simulink model "Sistema"  (R2023a)
settings: Solver=ode15s  StartTime=0.0  StopTime=10.0  MaxStep=1E-3  RelTol=1e-3
libraries: fl_lib x12, nesl_utility x6, ee_lib x2, slpidlib x1
settings Model: LastModifiedBy=osiri
settings DataIOCC: SaveFormat=Array  ReturnWorkspaceOutputs=off  TimeSaveName=t
settings DebuggingCC: AlgebraicLoopMsg=none  ArtificialAlgebraicLoopMsg=none  MaxConsecutiveZCsMsg=none  ModelReferenceExtraNoncontSigs=none  OperatingPointInterfaceChecksumMismatchMsg=none
settings RTWCC: GPUComputeCapability=5.0

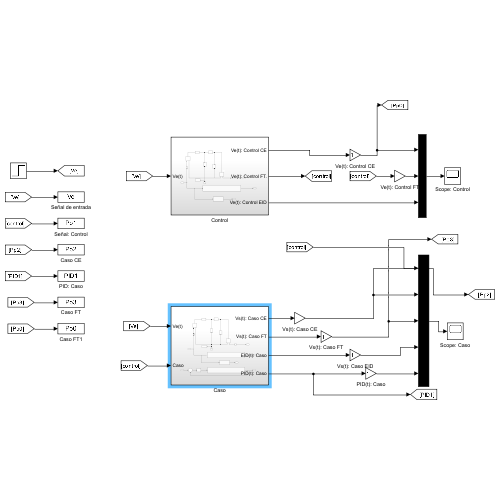
[thumbnail: Simulink's stored preview of the top-level diagram]
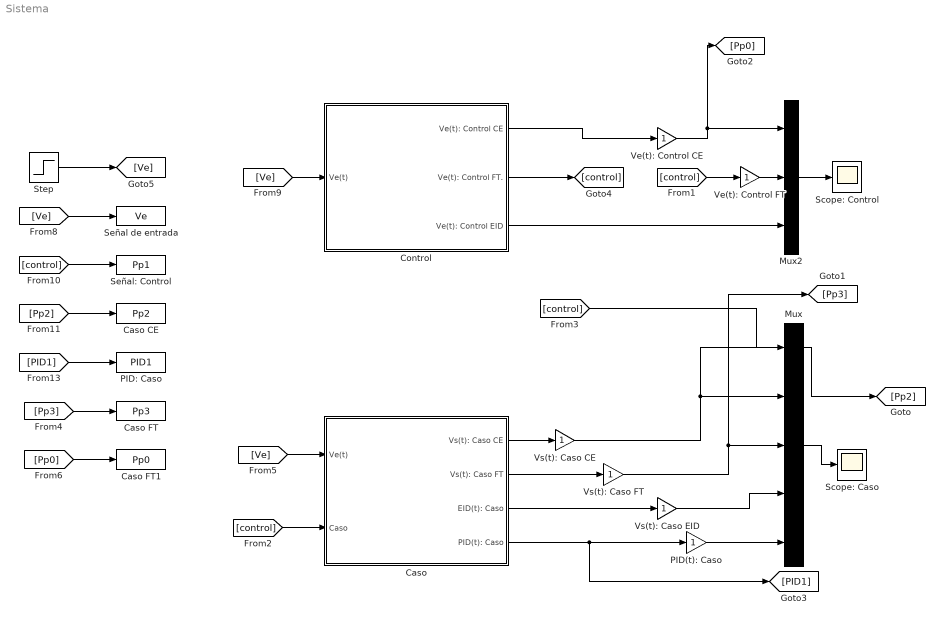
== system Sistema ==
  Caso : Subsystem
  Caso CE : ToWorkspace  VariableName=Pp2  SampleTime=-1
  Caso FT : ToWorkspace  VariableName=Pp3  SampleTime=-1
  Caso FT1 : ToWorkspace  VariableName=Pp0  SampleTime=-1
  Control : Subsystem
  Mux : Mux  Inputs=5
  Mux2 : Mux  Inputs=3
  PID(t): Caso : Gain
  PID: Caso : ToWorkspace  VariableName=PID1  SampleTime=-1
  Scope: Caso : Scope
  Scope: Control : Scope
  Señal de entrada : ToWorkspace  VariableName=Ve  SampleTime=-1
  Señal: Control : ToWorkspace  VariableName=Pp1  SampleTime=-1
  Step : Step  SampleTime=0
  Ve(t): Control CE : Gain
  Ve(t): Control FT : Gain
  Vs(t): Caso CE : Gain
  Vs(t): Caso EID : Gain
  Vs(t): Caso FT : Gain
  wires:
  Mux/1 -> Scope: Caso/1
  [control] -> Caso/2(Caso)
  [control] -> Mux/1
  Control/2(Ve(t): Control FT.) -> [control]
  Control/1(Ve(t): Control CE) -> Ve(t): Control CE/1
  Mux2/1 -> Scope: Control/1
  [Ve] -> Control/1(Ve(t))
  [control] -> Ve(t): Control FT/1
  [Ve] -> Señal de entrada/1
  [control] -> Señal: Control/1
  [Pp2] -> Caso CE/1
  [PID1] -> PID: Caso/1
  Step/1 -> [Ve]
  Ve(t): Control FT/1 -> Mux2/2
  Ve(t): Control CE/1 -> [Pp0], Mux2/1
  Vs(t): Caso CE/1 -> [Pp2], Mux/2
  Caso/1(Vs(t): Caso CE) -> Vs(t): Caso CE/1
  Vs(t): Caso FT/1 -> Mux/3, [Pp3]
  Caso/2(Vs(t): Caso FT) -> Vs(t): Caso FT/1
  Caso/4(PID(t): Caso) -> PID(t): Caso/1, [PID1]
  [Pp3] -> Caso FT/1
  [Pp0] -> Caso FT1/1
  Control/3(Ve(t): Control EID) -> Mux2/3
  PID(t): Caso/1 -> Mux/5
  Vs(t): Caso EID/1 -> Mux/4
  Caso/3(EID(t): Caso) -> Vs(t): Caso EID/1
  [Ve] -> Caso/1(Ve(t))

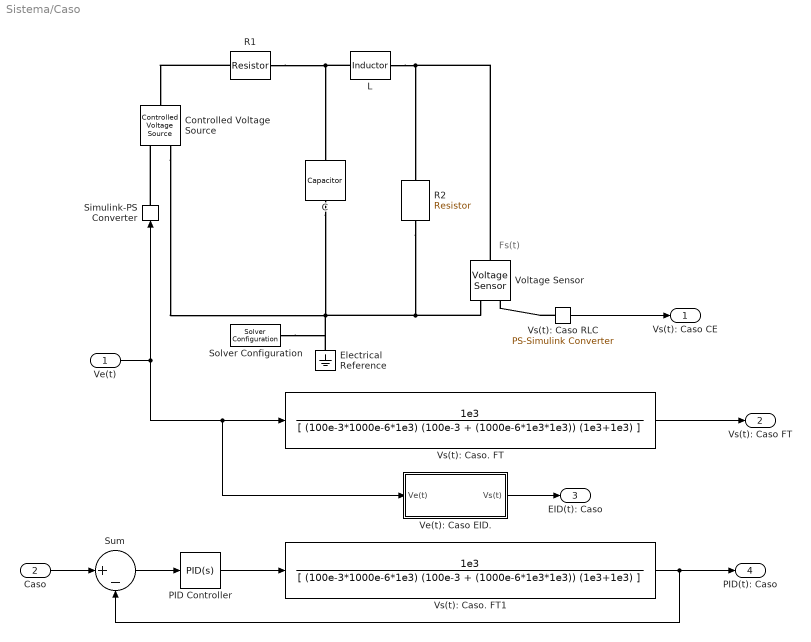
== system Sistema/Caso ==
  note: Fs(t)
  Ve(t) : Inport
  Caso : Inport  Port=2
  C : fl_lib/Electrical/Electrical Elements/Capacitor  c=1000e-6 F  r=1e-6 Ohm  g=0 1/Ohm  i_specify=off  i_priority=None  i=0 A  i_nominal_specify=off  i_nominal_unit=A  i_nominal_value=1  v_specify=off  v_priority=None  v=0 V  v_nominal_specify=off  v_nominal_unit=V  v_nominal_value=1  vc_specify=off  vc_priority=High  vc=0 V  vc_nominal_specify=off  vc_nominal_unit=V  vc_nominal_value=1
  Controlled Voltage Source : fl_lib/Electrical/Electrical Sources/Controlled Voltage Source
  Electrical Reference : fl_lib/Electrical/Electrical Elements/Electrical Reference
  L : ee_lib/Passive/Inductor  l=100e-3 H  enable_L_tol=ee.enum.toleranceApplication.none  L_tol=20  tol_distribution=ee.enum.toleranceDistribution.uniform  nSigma=4  r=0 Ohm  g=1e-9 1/Ohm  enable_operating_limits=ee.enum.enable.no  operating_limit_action=ee.enum.passive.reportOpLim.warn  max_working_current=1 A  power_rating=1 W  enable_faults=ee.enum.enable.no  fault_action=simscape.enum.assert.action.none  lambdaPercent=50  k_faulted=0.9999  turnsShort=ee.enum.passive.inductor.turnsShortOption.no  openCct=ee.enum.enable.no  groundShort=ee.enum.passive.inductor.groundShortOption.no  groundShortG=0 1/Ohm  tau_fault=1e-3 s  fault_trigger=ee.enum.faults.faultTrigger.temporal  t_fault=1 s  max_permissible_voltage=100 V  n_fail_on_voltage=1  max_permissible_current=1 A  t_fail_on_current=1 s  i_L_specify=off  i_L_priority=High  i_L=0 A  i_L_nominal_specify=off  i_L_nominal_unit=A  i_L_nominal_value=1
  PID Controller : slpidlib/PID Controller  Controller=PID  Form=Parallel  TimeDomain=Continuous-time  UseExternalTs=off  SampleTime=-1  IntegratorMethod=Forward Euler  FilterMethod=Forward Euler  ControllerParametersSource=internal  P=132.81296326735  I=3266.13831963624  UseKiTs=off  D=0.180716891182534  N=507.693883251119  UseFilter=on  TunerSelectOption=Transfer Function Based (PID Tuner App)  InitialConditionSource=internal  InitialConditionForIntegrator=0  InitialConditionForFilter=0  DifferentiatorICPrevScaledInput=0  ExternalReset=none  TrackingMode=off  Kt=1  LimitOutput=off  SatLimitsSource=internal  UpperSaturationLimit=inf  LowerSaturationLimit=-inf  LinearizeAsGain=on  AntiWindupMode=none  Kb=1  LimitIntegrator=off  UpperIntegratorSaturationLimit=inf  LowerIntegratorSaturationLimit=-inf  POutMin=[]  POutMax=[]  IOutMin=[]  IOutMax=[]  DOutMin=[]  DOutMax=[]  NOutMin=[]  NOutMax=[]  SumOutMin=[]  SumOutMax=[]  SaturationOutMin=[]  SaturationOutMax=[]  PParamMin=[]  PParamMax=[]  IParamMin=[]  IParamMax=[]  DParamMin=[]  DParamMax=[]  NParamMin=[]  NParamMax=[]  KbParamMin=[]  KbParamMax=[]  KtParamMin=[]  KtParamMax=[]  KbOutMin=[]  KbOutMax=[]  KtOutMin=[]  KtOutMax=[]  IntegratorOutMin=[]  IntegratorOutMax=[]  FilterOutMin=[]  FilterOutMax=[]  SumI1OutMin=[]  SumI1OutMax=[]  SumI2OutMin=[]  SumI2OutMax=[]  SumI3OutMin=[]  SumI3OutMax=[]  SumI4OutMin=[]  SumI4OutMax=[]  SumDOutMin=[]  SumDOutMax=[]  DifferentiatorOutMin=[]  DifferentiatorOutMax=[]  FilterDiffOutCoefMin=[]  FilterDiffOutCoefMax=[]  ReciprocalOutMin=[]  ReciprocalOutMax=[]  SumDenOutMin=[]  SumDenOutMax=[]  SumNumOutMin=[]  SumNumOutMax=[]  DivideOutMin=[]  DivideOutMax=[]  UdiffTsProdOutMin=[]  UdiffTsProdOutMax=[]  NTsProdOutMin=[]  NTsProdOutMax=[]  UintegralTsProdOutMin=[]  UintegralTsProdOutMax=[]  UngainTsProdOutMin=[]  UngainTsProdOutMax=[]  ClampingZeroOutDataTypeStr=Inherit: Inherit via back propagation  ClampingZeroOutMin=[]  ClampingZeroOutMax=[]  FilterDenConstantOutDataTypeStr=Inherit: Inherit via back propagation  FilterDenConstantOutMin=[]  FilterDenConstantOutMax=[]  PCopyOutDataTypeStr=Inherit: Inherit via back propagation  PCopyOutMin=[]  PCopyOutMax=[]  NCopyOutDataTypeStr=Inherit: Inherit via back propagation  NCopyOutMin=[]  NCopyOutMax=[]  IntegratorContinuousStateAttributes=''  IntegratorStateMustResolveToSignalObject=off  IntegratorRTWStateStorageClass=Auto  FilterContinuousStateAttributes=''  FilterStateMustResolveToSignalObject=off  FilterRTWStateStorageClass=Auto  ParallelPVariant=InternalParameters  IdealPVariant=Disabled  IVariant=InternalParameters  DVariant=InternalParameters  IntegratorVariant=Continuous  SatVariant=Disabled  AWVariant=Passthrough  PCopyVariant=Disabled  TRVariant=Disabled  FdbkBlocksVariant=Forward  IdealPFdbkVariant=Disabled  SatFdbkVariant=Disabled  DerivativeFilterVariant=ContFilter  NVariant=InternalParameters  NCopyVariant=Disabled  FilterICVariant=InternalICsFilter  IntegratorICVariant=InternalICs  ExternalResetVariant=Disabled  TRSumVariant=Passthrough  SumFdbkVariant=Disabled  SumVariant=Sum_PID  TsampFilterVariant=InternalTs  TsampNgainVariant=Passthrough  TsampIntegralVariant=Disabled_SignalSpec  ExternalSaturationOutDataTypeStr=Inherit: Same as second input
  R1 : fl_lib/Electrical/Electrical Elements/Resistor  R=1e3 Ohm  i_specify=off  i_priority=None  i=0 A  i_nominal_specify=off  i_nominal_unit=A  i_nominal_value=1  v_specify=off  v_priority=None  v=0 V  v_nominal_specify=off  v_nominal_unit=V  v_nominal_value=1
  R2 : fl_lib/Electrical/Electrical Elements/Resistor  R=1e3 Ohm  i_specify=off  i_priority=None  i=0 A  i_nominal_specify=off  i_nominal_unit=A  i_nominal_value=1  v_specify=off  v_priority=None  v=0 V  v_nominal_specify=off  v_nominal_unit=V  v_nominal_value=1
  Simulink-PS Converter : nesl_utility/Simulink-PS Converter  PhysicalDomain=network_engine_domain  SubClassName=ps_input  LeftPortType=input  RightPortType=output  PseudoPeriodic=off  Frequencies=[]  NoiseDistribution=none  NoiseParameters=[]  Unit=1  AffineConversion=off  FilteringAndDerivatives=provide  SimscapeFilterOrder=1  InputFilterTimeConstant=0.001  UdotUserProvided=0
  Solver Configuration : nesl_utility/Solver Configuration  PhysicalDomain=network_engine_domain  SubClassName=solver  LeftPortType=input  RightPortType=generic  Tones=[]  Harmonics=[]  SimulateNoise=off  Profile=off  UseLocalSampling=off  EnableSwitchedLinearOptims=on  FrequencyDomain=off  UseCCode=off  RelTol=0.001  AbsTol=0.001  MinStep=1e-09  ToWorkspace=off  RevertToSquareIcSolve=off  NumHomotopyIterations=100  PhasorMode=off  PhasorModeNumHarmonics=1  ConsistencySolver=NEWTON_XTOL_AFTER_FTOL  IndexReductionMethod=DerivativeReplacement  DoDC=off  ResidualTolerance=1e-09  ConsistencyTolSource=GLOBAL  ConsistencyAbsTol=0.001  ConsistencyRelTol=0.001  ConsistencyTolFactor=0.001  UseLocalSolver=off  LocalSolverChoice=NE_BACKWARD_EULER_ADVANCER  ResolveIndetEquations=on  FunctionEvalNumThread=1  LocalSolverSampleTime=0.001  DoFixedCost=off  MaxNonlinIter=3  MaxModeIter=2  ComputeImpulses=off  ImpulseIterations=2  LinearAlgebra=auto  LinearAlgebraNumThread=0  EquationFormulation=NE_TIME_EF  DelaysMemoryBudget=1024  AutomaticFiltering=on  FilteringTimeConstant=0.001  PartitionStorageMethod=AS_NEEDED  PartitionMemoryBudget=1024  PartitionMethod=ROBUST
  Sum : Sum  Inputs=|+-
  Ve(t): Caso EID. : Subsystem
  Voltage Sensor : fl_lib/Electrical/Electrical Sensors/Voltage Sensor
  Vs(t): Caso RLC : nesl_utility/PS-Simulink Converter  PhysicalDomain=network_engine_domain  SubClassName=ps_output  LeftPortType=input  RightPortType=output  PseudoPeriodic=off  Frequencies=[]  VectorFormat=1-D array  Unit=inherit  AffineConversion=off
  Vs(t): Caso. FT : TransferFcn  Numerator=[1e3]  Denominator=[ (100e-3*1000e-6*1e3) (100e-3 + (1000e-6*1e3*1e3)) (1e3+1e3) ]
  Vs(t): Caso. FT1 : TransferFcn  Numerator=[1e3]  Denominator=[ (100e-3*1000e-6*1e3) (100e-3 + (1000e-6*1e3*1e3)) (1e3+1e3) ]
  Vs(t): Caso CE : Outport
  Vs(t): Caso FT : Outport  Port=2
  EID(t): Caso : Outport  Port=3
  PID(t): Caso : Outport  Port=4
  wires:
  Sum/1 -> PID Controller/1
  Vs(t): Caso. FT1/1 -> PID(t): Caso/1, Sum/2
  PID Controller/1 -> Vs(t): Caso. FT1/1
  Caso/1 -> Sum/1
  Vs(t): Caso RLC/1 -> Vs(t): Caso CE/1
  Ve(t)/1 -> Ve(t): Caso EID./1(Ve(t)), Vs(t): Caso. FT/1, Simulink-PS Converter/1
  Vs(t): Caso. FT/1 -> Vs(t): Caso FT/1
  Ve(t): Caso EID./1(Vs(t)) -> EID(t): Caso/1
  connections:
  R1/LConn1 -- C/LConn1 -- L/LConn1
  Voltage Sensor/RConn2 -- Solver Configuration/RConn1 -- Electrical Reference/LConn1 -- C/RConn1 -- Controlled Voltage Source/RConn2 -- R2/LConn1
  Simulink-PS Converter/RConn1 -- Controlled Voltage Source/RConn1
  R1/RConn1 -- Controlled Voltage Source/LConn1
  Vs(t): Caso RLC/LConn1 -- Voltage Sensor/RConn1
  L/RConn1 -- Voltage Sensor/LConn1 -- R2/RConn1

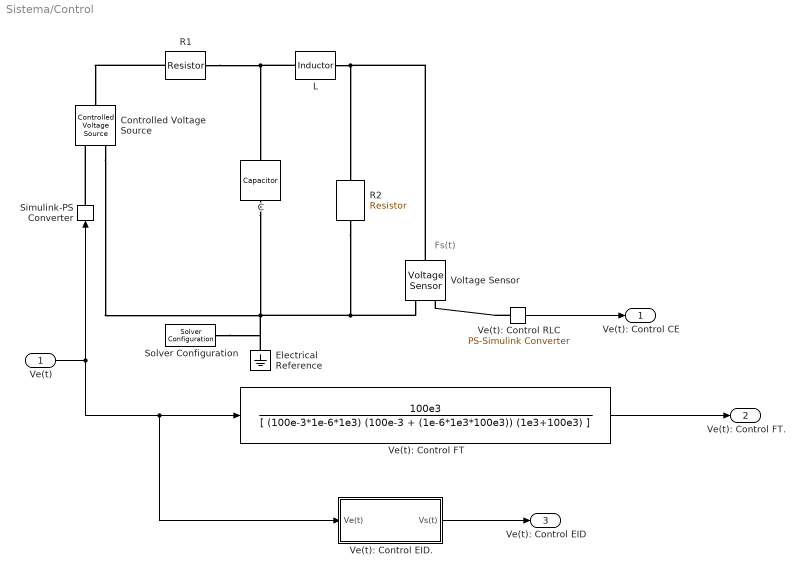
== system Sistema/Control ==
  note: Fs(t)
  Ve(t) : Inport
  C : fl_lib/Electrical/Electrical Elements/Capacitor  c=1e-6 F  r=1e-6 Ohm  g=0 1/Ohm  i_specify=off  i_priority=None  i=0 A  i_nominal_specify=off  i_nominal_unit=A  i_nominal_value=1  v_specify=off  v_priority=None  v=0 V  v_nominal_specify=off  v_nominal_unit=V  v_nominal_value=1  vc_specify=off  vc_priority=High  vc=0 V  vc_nominal_specify=off  vc_nominal_unit=V  vc_nominal_value=1
  Controlled Voltage Source : fl_lib/Electrical/Electrical Sources/Controlled Voltage Source
  Electrical Reference : fl_lib/Electrical/Electrical Elements/Electrical Reference
  L : ee_lib/Passive/Inductor  l=100e-3 H  enable_L_tol=ee.enum.toleranceApplication.none  L_tol=20  tol_distribution=ee.enum.toleranceDistribution.uniform  nSigma=4  r=0 Ohm  g=1e-9 1/Ohm  enable_operating_limits=ee.enum.enable.no  operating_limit_action=ee.enum.passive.reportOpLim.warn  max_working_current=1 A  power_rating=1 W  enable_faults=ee.enum.enable.no  fault_action=simscape.enum.assert.action.none  lambdaPercent=50  k_faulted=0.9999  turnsShort=ee.enum.passive.inductor.turnsShortOption.no  openCct=ee.enum.enable.no  groundShort=ee.enum.passive.inductor.groundShortOption.no  groundShortG=0 1/Ohm  tau_fault=1e-3 s  fault_trigger=ee.enum.faults.faultTrigger.temporal  t_fault=1 s  max_permissible_voltage=100 V  n_fail_on_voltage=1  max_permissible_current=1 A  t_fail_on_current=1 s  i_L_specify=off  i_L_priority=High  i_L=0 A  i_L_nominal_specify=off  i_L_nominal_unit=A  i_L_nominal_value=1
  R1 : fl_lib/Electrical/Electrical Elements/Resistor  R=1e3 Ohm  i_specify=off  i_priority=None  i=0 A  i_nominal_specify=off  i_nominal_unit=A  i_nominal_value=1  v_specify=off  v_priority=None  v=0 V  v_nominal_specify=off  v_nominal_unit=V  v_nominal_value=1
  R2 : fl_lib/Electrical/Electrical Elements/Resistor  R=100e3 Ohm  i_specify=off  i_priority=None  i=0 A  i_nominal_specify=off  i_nominal_unit=A  i_nominal_value=1  v_specify=off  v_priority=None  v=0 V  v_nominal_specify=off  v_nominal_unit=V  v_nominal_value=1
  Simulink-PS Converter : nesl_utility/Simulink-PS Converter  PhysicalDomain=network_engine_domain  SubClassName=ps_input  LeftPortType=input  RightPortType=output  PseudoPeriodic=off  Frequencies=[]  NoiseDistribution=none  NoiseParameters=[]  Unit=1  AffineConversion=off  FilteringAndDerivatives=provide  SimscapeFilterOrder=1  InputFilterTimeConstant=0.001  UdotUserProvided=0
  Solver Configuration : nesl_utility/Solver Configuration  PhysicalDomain=network_engine_domain  SubClassName=solver  LeftPortType=input  RightPortType=generic  Tones=[]  Harmonics=[]  SimulateNoise=off  Profile=off  UseLocalSampling=off  EnableSwitchedLinearOptims=on  FrequencyDomain=off  UseCCode=off  RelTol=0.001  AbsTol=0.001  MinStep=1e-09  ToWorkspace=off  RevertToSquareIcSolve=off  NumHomotopyIterations=100  PhasorMode=off  PhasorModeNumHarmonics=1  ConsistencySolver=NEWTON_XTOL_AFTER_FTOL  IndexReductionMethod=DerivativeReplacement  DoDC=off  ResidualTolerance=1e-09  ConsistencyTolSource=GLOBAL  ConsistencyAbsTol=0.001  ConsistencyRelTol=0.001  ConsistencyTolFactor=0.001  UseLocalSolver=off  LocalSolverChoice=NE_BACKWARD_EULER_ADVANCER  ResolveIndetEquations=on  FunctionEvalNumThread=1  LocalSolverSampleTime=0.001  DoFixedCost=off  MaxNonlinIter=3  MaxModeIter=2  ComputeImpulses=off  ImpulseIterations=2  LinearAlgebra=auto  LinearAlgebraNumThread=0  EquationFormulation=NE_TIME_EF  DelaysMemoryBudget=1024  AutomaticFiltering=on  FilteringTimeConstant=0.001  PartitionStorageMethod=AS_NEEDED  PartitionMemoryBudget=1024  PartitionMethod=ROBUST
  Ve(t): Control EID. : Subsystem
  Ve(t): Control FT : TransferFcn  Numerator=[100e3]  Denominator=[ (100e-3*1e-6*1e3) (100e-3 + (1e-6*1e3*100e3)) (1e3+100e3) ]
  Ve(t): Control RLC : nesl_utility/PS-Simulink Converter  PhysicalDomain=network_engine_domain  SubClassName=ps_output  LeftPortType=input  RightPortType=output  PseudoPeriodic=off  Frequencies=[]  VectorFormat=1-D array  Unit=inherit  AffineConversion=off
  Voltage Sensor : fl_lib/Electrical/Electrical Sensors/Voltage Sensor
  Ve(t): Control CE : Outport
  Ve(t): Control FT. : Outport  Port=2
  Ve(t): Control EID : Outport  Port=3
  wires:
  Ve(t): Control FT/1 -> Ve(t): Control FT./1
  Ve(t): Control RLC/1 -> Ve(t): Control CE/1
  Ve(t)/1 -> Ve(t): Control EID./1(Ve(t)), Ve(t): Control FT/1, Simulink-PS Converter/1
  Ve(t): Control EID./1(Vs(t)) -> Ve(t): Control EID/1
  connections:
  Simulink-PS Converter/RConn1 -- Controlled Voltage Source/RConn1
  Voltage Sensor/RConn2 -- R2/LConn1 -- Solver Configuration/RConn1 -- Electrical Reference/LConn1 -- C/RConn1 -- Controlled Voltage Source/RConn2
  Ve(t): Control RLC/LConn1 -- Voltage Sensor/RConn1
  R1/RConn1 -- Controlled Voltage Source/LConn1
  R1/LConn1 -- L/LConn1 -- C/LConn1
  L/RConn1 -- Voltage Sensor/LConn1 -- R2/RConn1

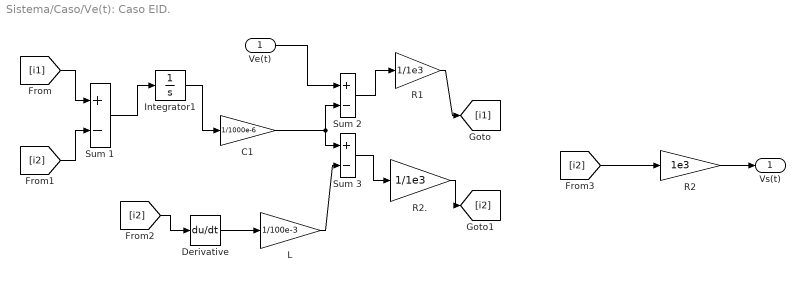
== system Sistema/Caso/Ve(t): Caso EID. ==
  Ve(t) : Inport
  C1 : Gain  Gain=1/1000e-6
  Derivative : Derivative
  Integrator1 : Integrator
  L : Gain  Gain=1/100e-3
  R1 : Gain  Gain=1/1e3
  R2 : Gain  Gain=1e3
  R2. : Gain  Gain=1/1e3
  Sum 1 : Sum  Inputs=+-
  Sum 2 : Sum  Inputs=+-
  Sum 3 : Sum  Inputs=+-
  Vs(t) : Outport
  wires:
  R2/1 -> Vs(t)/1
  [i1] -> Sum 1/1
  [i2] -> Sum 1/2
  Sum 1/1 -> Integrator1/1
  Integrator1/1 -> C1/1
  Ve(t)/1 -> Sum 2/1
  C1/1 -> Sum 3/1, Sum 2/2
  Sum 2/1 -> R1/1
  R1/1 -> [i1]
  L/1 -> Sum 3/2
  Derivative/1 -> L/1
  [i2] -> Derivative/1
  Sum 3/1 -> R2./1
  R2./1 -> [i2]
  [i2] -> R2/1

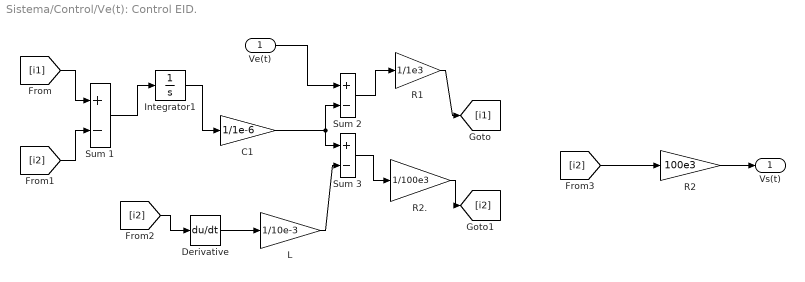
== system Sistema/Control/Ve(t): Control EID. ==
  Ve(t) : Inport
  C1 : Gain  Gain=1/1e-6
  Derivative : Derivative
  Integrator1 : Integrator
  L : Gain  Gain=1/10e-3
  R1 : Gain  Gain=1/1e3
  R2 : Gain  Gain=100e3
  R2. : Gain  Gain=1/100e3
  Sum 1 : Sum  Inputs=+-
  Sum 2 : Sum  Inputs=+-
  Sum 3 : Sum  Inputs=+-
  Vs(t) : Outport
  wires:
  R2/1 -> Vs(t)/1
  [i1] -> Sum 1/1
  [i2] -> Sum 1/2
  Sum 1/1 -> Integrator1/1
  Integrator1/1 -> C1/1
  Ve(t)/1 -> Sum 2/1
  C1/1 -> Sum 3/1, Sum 2/2
  Sum 2/1 -> R1/1
  R1/1 -> [i1]
  L/1 -> Sum 3/2
  Derivative/1 -> L/1
  [i2] -> Derivative/1
  Sum 3/1 -> R2./1
  R2./1 -> [i2]
  [i2] -> R2/1
